simulink model "water_heatOfTank"  (R2024b)
settings: Solver=VariableStepAuto  StartTime=0.0  StopTime=10.0  RelTol=1e-3
settings Model: Creator=ksamb  LastModifiedBy=ksamb

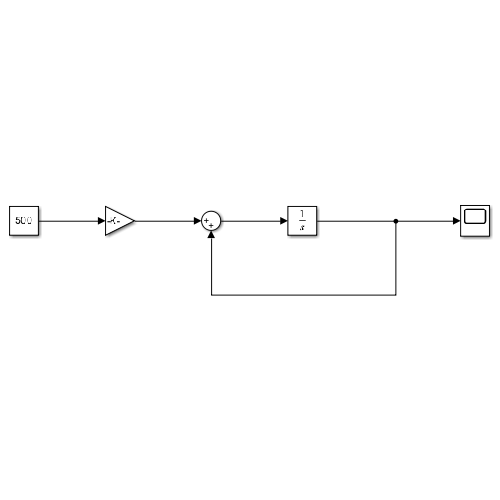
[thumbnail: Simulink's stored preview of the top-level diagram]
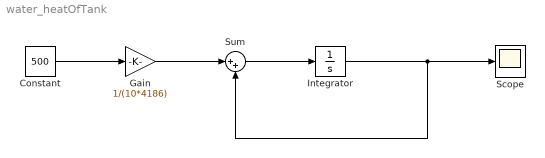
== system water_heatOfTank ==
  Constant : Constant  Value=500
  Gain : Gain  Gain=1/(10*4186)
  Integrator : Integrator  InitialCondition=20
  Scope : Scope
  Sum : Sum  Inputs=|++
  wires:
  Constant/1 -> Gain/1
  Sum/1 -> Integrator/1
  Integrator/1 -> Sum/2, Scope/1
  Gain/1 -> Sum/1
